simulink model "untitled"  (R2016a)
settings: Solver=VariableStepAuto  StartTime=0.0  StopTime=10.0  RelTol=1e-3
libraries: simulink x1
settings Model: Creator=Student  LastModifiedBy=Student

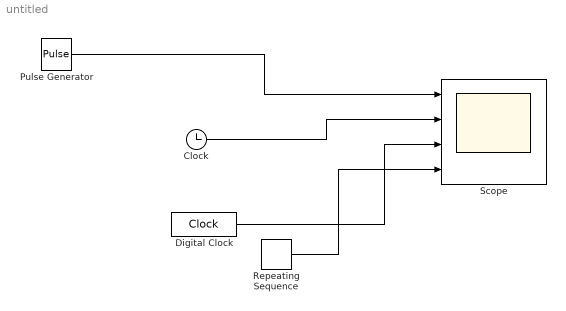
== system untitled ==
  Clock : Clock
  Digital Clock : DigitalClock
  Pulse Generator : DiscretePulseGenerator  PulseType=Time based  Period=10  PulseWidth=5
  Repeating Sequence : simulink/Sources/Repeating Sequence  rep_seq_t=[0 5]  rep_seq_y=[0 5]
  Scope : Scope  NumInputPorts=4
  wires:
  Pulse Generator/1 -> Scope/1
  Clock/1 -> Scope/2
  Digital Clock/1 -> Scope/3
  Repeating Sequence/1 -> Scope/4
